simulink model "RBCM_Model"  (R2024b)
settings: Solver=FixedStepAuto  StartTime=0.0  StopTime=10.0  RelTol=1e-3
PreLoadFcn:
  | % NXP_MBDT_S32K3 callback: DO NOT REMOVE
  | mbd_s32k3.common.nxp.model_callbacks.preLoadFcn();
PostLoadFcn:
  | % NXP_MBDT_S32K3 callback: DO NOT REMOVE
  | mbd_s32k3.common.nxp.model_callbacks.postLoadFcn();
InitFcn:
  | % NXP_MBDT_S32K3 callback: DO NOT REMOVE
  | mbd_s32k3.common.nxp.model_callbacks.initFcn();
undefined symbols (not defined in the file or in its folder): AccuFanPwr_hHsd3ch2, BspdPwr_lHsd1ch2, BuzzerPwr_lHsd3ch3, DevicePwr_12v_lHsd1ch1, DevicePwr_hHsd1ch2, DrsPwr_8v_lHsd3ch1, hHsd_Diagnose_AdcBuffer, ILPwr_hHsd1ch1, lHsd_Diagnose_AdcBuffer, LoggerPwr_lHsd1ch3, PumpFan1_hHsd4ch1, PumpFan2_hHsd4ch2, PumpPwr_hHsd3ch1, RGBLED0state, TaillightPwr_lHsd3ch4, TempSensorPwr_lHsd1ch4
libraries: mbd_s32k3_io_library x127, simulink x48, canmsglib x8, mbd_s32k3_communication_library x7, mbd_s32k3_isr_library x6, mbd_s32k3_cdd_library x3, mbd_s32k3_utility_library x1
(part 6 of 10)

== system RBCM_Model/错误码数据发送(未)1 ==
  Trigger : TriggerPort  TriggerType=function-call  VariantControl=(inherit)  PortDimensions=1
  Bus Selector : BusSelector  OutputSignals=Data,Length,ID
  CAN Pack : canmsglib/CAN Pack  CANdbFile=E:\Workspace\Myworkspace\RBCM_S32K344_AUTOSAR_MBD\Firmware\AUTOSAR_MBD\RBCM_ModelConfig\E10_dbc_240819_CAN.dbc  MsgList=RBCM_Diagnose_Data  MsgName=RBCM_Diagnose_Data  MsgIDType=Extended (29-bit identifier)  MsgIdentifier=252996466  CANIDInput=off  MsgLength=2  Remote=off  ApplyMinMax=off  BusOutput=on  SignalInfo={'PDB_Error_Device','0','8','LE','unsigned','Standard','0','1','0','-Inf','Inf';'PDB_Error_State','8','8','LE','unsigned','Standard','0','1','0','-Inf','Inf'}
      settings: LibrarySourceBlock=canlib/CAN Pack  DataFormat=CANdb specified signals
  Can : mbd_s32k3_communication_library/Can  api_func=Can_Write  controller=No controller configured  hw_obj=CanHardwareObject_Can0_Tx_Interrupt  mode=CAN_CS_STARTED  canfd_msg=off  ext_id_msg=off  empty_msg=off  text=|
      | CanConfigSet - CanConfigSet 
      | CanConfigSet/CanController - CanController_0 
      | CanConfigSet/CanController_0/CanAutoBusOffRecovery - false 
      | CanConfigSet/CanController_0/CanBusoffProcessing - POLLING 
      | CanConfigSet/CanController_0/CanControllerActivation - true 
      | CanConfigSet/CanController_0/CanControllerBaseAddress - 0 
      | CanConfigSet/CanController_0/CanControllerBaudrateConfig - CanControllerBaudrateConfig_0 
      | CanConfigSet/CanController_0/CanControllerBaudrateConfig_0/CanAdvancedSetting - false 
      | CanConfigSet/CanController_0/CanControllerBaudrateConfig_0/CanBaudrateTypeSuport - NORMAL_CBT 
      | CanConfigSet/CanController_0/CanControllerBaudrateConfig_0/CanBusLength - 40 
      | CanConfigSet/CanController_0/CanControllerBaudrateConfig_0/CanControllerBaudRate - 500.0 
      | CanConfigSet/CanController_0/CanControllerBaudrateConfig_0/CanControllerBaudRateConfigID - 0 
      | CanConfigSet/CanController_0/CanControllerBaudrateConfig_0/CanControllerFdBaudrateConfig - CanControllerFdBaudrateConfig 
      | CanConfigSet/CanController_0/CanControllerBaudrateConfig_0/CanControllerFdBaudrateConfig/CanControllerFdBaudRate - 2000 
      | CanConfigSet/CanController_0/CanControllerBaudrateConfig_0/CanControllerFdBaudrateConfig/CanControllerFdPrescaller - 2 
      | CanConfigSet/CanController_0/CanControllerBaudrateConfig_0/CanControllerFdBaudrateConfig/CanControllerFdSyncSeg - 1 
      | CanConfigSet/CanController_0/CanControllerBaudrateConfig_0/CanControllerFdBaudrateConfig/CanControllerPrescallerAlternateFd - 1 
      | CanConfigSet/CanController_0/CanControllerBaudrateConfig_0/CanControllerFdBaudrateConfig/CanControllerPropSeg - 5 
      | CanConfigSet/CanController_0/CanControllerBaudrateConfig_0/CanControllerFdBaudrateConfig/CanControllerSeg1 - 2 
      | CanConfigSet/CanController_0/CanControllerBaudrateConfig_0/CanControllerFdBaudrateConfig/CanControllerSeg2 - 2 
      | CanConfigSet/CanController_0/CanControllerBaudrateConfig_0/CanControllerFdBaudrateConfig/CanControllerSyncJumpWidth - 2 
      | CanConfigSet/CanController_0/CanControllerBaudrateConfig_0/CanControllerFdBaudrateConfig/CanControllerTxBitRateSwitch - true 
      | CanConfigSet/CanController_0/CanControllerBaudrateConfig_0/CanControllerFdBaudrateConfig/Index - 0 
      | CanConfigSet/CanController_0/CanControllerBaudrateConfig_0/CanControllerPrescaller - 2 
      | CanConfigSet/CanController_0/CanControllerBaudrateConfig_0/CanControllerPrescallerAlternate - 10 
      | CanConfigSet/CanController_0/CanControllerBaudrateConfig_0/CanControllerPropSeg - 11 
      | CanConfigSet/CanController_0/CanControllerBaudrateConfig_0/CanControllerSeg1 - 18 
      | CanConfigSet/CanController_0/CanControllerBaudrateConfig_0/CanControllerSeg2 - 10 
      | CanConfigSet/CanController_0/CanControllerBaudrateConfig_0/CanControllerSyncJumpWidth - 10 
      | CanConfigSet/CanController_0/CanControllerBaudrateConfig_0/CanControllerSyncSeg - 1 
      | CanConfigSet/CanController_0/CanControllerBaudrateConfig_0/CanPropDelayTranceiver - 150.0 
      | CanConfigSet/CanController_0/CanControllerBaudrateConfig_0/CanTxArbitrationStartDelay - 12 
      | CanConfigSet/CanController_0/CanControllerBaudrateConfig_0/Index - 0 
      | CanConfigSet/CanController_0/CanControllerDefaultBaudrate - /Can_43_FLEXCAN/Can/CanConfigSet/CanController_0/CanControllerBaudrateConfig_0 
      | CanConfigSet/CanController_0/CanControllerEdgeFilter - false 
      | CanConfigSet/CanController_0/CanControllerFdISO - true 
      | CanConfigSet/CanController_0/CanControllerId - 0 
      | CanConfigSet/CanController_0/CanControllerPrExcEn - false 
      | CanConfigSet/CanController_0/CanCpuClockRef - /Mcu/Mcu/McuModuleConfiguration/McuClockSettingConfig_0/FLEXCAN_PE_CLK0_2 
      | CanConfigSet/CanController_0/CanCpuClockRefAlternate - /Mcu/Mcu/McuModuleConfiguration/McuClockSettingConfig_0/FLEXCAN_PE_CLK0_2 
      | CanConfigSet/CanController_0/CanHwChannel - FLEXCAN_0 
      | CanConfigSet/CanController_0/CanLoopBackMode - false 
      | CanConfigSet/CanController_0/CanRamBlock - CanRamBlock 
      | CanConfigSet/CanController_0/CanRamBlock/CanRamBlockUnified - CanRamBlockUnified 
      | CanConfigSet/CanController_0/CanRamBlock/CanRamBlockUnified/CanBlockUnifiedPayloadLength - CAN_16_BYTES_PAYLOAD 
      | CanConfigSet/CanController_0/CanRamBlock/Choice - CanRamBlockUnified 
      | CanConfigSet/CanController_0/CanRamBlock/Index - 0 
      | CanConfigSet/CanController_0/CanRxFiFo - CanRxFiFo 
      | CanConfigSet/CanController_0/CanRxFiFo/CanEnhanceFiFo - CanRxFiFo 
      | CanConfigSet/CanController_0/CanRxFiFo/CanRxFiFo/CanEnhanceFiFoDmaEnable - false 
      | CanConfigSet/CanController_0/CanRxFiFo/CanRxFiFo/CanEnhancedSchemeType - MASK_FILTER_SCHEME 
      | CanConfigSet/CanController_0/CanRxFiFo/CanRxFiFo/CanFiFoDmaErrorNotif - NULL_PTR 
      | CanConfigSet/CanController_0/CanRxFiFo/CanRxFiFo/CanFiFoOverflowNotif - MBDT_FlexCAN0_FifoOverflowNotif 
      | CanConfigSet/CanController_0/CanRxFiFo/CanRxFiFo/NumberMBTransferDMA - 1 
      | CanConfigSet/CanController_0/CanRxFiFo/Choice - CanEnhanceFiFo 
      | CanConfigSet/CanController_0/CanRxFiFo/Index - 0 
      | CanConfigSet/CanController_0/CanRxProcessing - MIXED 
      | CanConfigSet/CanController_0/CanTrippleSamplingEnable - false 
      | CanConfigSet/CanController_0/CanTxProcessing - MIXED 
      | CanConfigSet/CanController_0/CanWakeupFunctionalityAPI - false 
      | CanConfigSet/CanController_0/CanWakeupProcessing - POLLING 
      | CanConfigSet/CanController_0/CanWakeupSupport - false 
      | CanConfigSet/CanController_0/Index - 0 
      | CanConfigSet/CanHardwareObject - CanHardwareObject_Can0_Rx_Ext_Interrupt CanHardwareObject_Can0_Rx_FIFO CanHardwareObject_Can0_Rx_Std_Polling CanHardwareObject_Can0_Tx_Interrupt CanHardwareObject_Can0_Tx_Polling 
      | CanConfigSet/CanHardwareObject_Can0_Rx_Ext_Interrupt/CanControllerRef - /Can_43_FLEXCAN/Can/CanConfigSet/CanController_0 
      | CanConfigSet/CanHardwareObject_Can0_Rx_Ext_Interrupt/CanHandleType - BASIC 
      | CanConfigSet/CanHardwareObject_Can0_Rx_Ext_Interrupt/CanHardwareObjectUsesPolling - false 
      | CanConfigSet/CanHardwareObject_Can0_Rx_Ext_Interrupt/CanHwFilter - CanHwFilter_0 
      | CanConfigSet/CanHardwareObject_Can0_Rx_Ext_Interrupt/CanHwFilter_0/CanHwFilterCode - 0 
      | CanConfigSet/CanHardwareObject_Can0_Rx_Ext_Interrupt/CanHwFilter_0/CanHwFilterMask - 0 
      | CanConfigSet/CanHardwareObject_Can0_Rx_Ext_Interrupt/CanHwFilter_0/Index - 0 
      | CanConfigSet/CanHardwareObject_Can0_Rx_Ext_Interrupt/CanHwObjectCount - 1 
      | CanConfigSet/CanHardwareObject_Can0_Rx_Ext_Interrupt/CanIdType - EXTENDED 
      | CanConfigSet/CanHardwareObject_Can0_Rx_Ext_Interrupt/CanObjectId - 2 
      | CanConfigSet/CanHardwareObject_Can0_Rx_Ext_Interrupt/CanObjectType - RECEIVE 
      | CanConfigSet/CanHardwareObject_Can0_Rx_Ext_Interrupt/Index - 2 
      | CanConfigSet/CanHardwareObject_Can0_Rx_FIFO/CanControllerRef - /Can_43_FLEXCAN/Can/CanConfigSet/CanController_0 
      | CanConfigSet/CanHardwareObject_Can0_Rx_FIFO/CanHandleType - BASIC 
      | CanConfigSet/CanHardwareObject_Can0_Rx_FIFO/CanHardwareObjectUsesPolling - false 
      | CanConfigSet/CanHardwareObject_Can0_Rx_FIFO/CanHwFilter - CanHwFilter_0 CanHwFilter_1 CanHwFilter_2 CanHwFilter_3 CanHwFilter_4 CanHwFilter_5 CanHwFilter_6 CanHwFilter_7 
      | CanConfigSet/CanHardwareObject_Can0_Rx_FIFO/CanHwFilter_0/CanHwFilterCode - 1008 
      | CanConfigSet/CanHardwareObject_Can0_Rx_FIFO/CanHwFilter_0/CanHwFilterMask - 536870911 
      | CanConfigSet/CanHardwareObject_Can0_Rx_FIFO/CanHwFilter_0/Index - 0 
      | CanConfigSet/CanHardwareObject_Can0_Rx_FIFO/CanHwFilter_1/CanHwFilterCode - 1009 
      | CanConfigSet/CanHardwareObject_Can0_Rx_FIFO/CanHwFilter_1/CanHwFilterMask - 536870911 
      | CanConfigSet/CanHardwareObject_Can0_Rx_FIFO/CanHwFilter_1/Index - 1 
      | CanConfigSet/CanHardwareObject_Can0_Rx_FIFO/CanHwFilter_2/CanHwFilterCode - 1010 
      | CanConfigSet/CanHardwareObject_Can0_Rx_FIFO/CanHwFilter_2/CanHwFilterMask - 536870911 
      | CanConfigSet/CanHardwareObject_Can0_Rx_FIFO/CanHwFilter_2/Index - 2 
      | CanConfigSet/CanHardwareObject_Can0_Rx_FIFO/CanHwFilter_3/CanHwFilterCode - 1011 
      | CanConfigSet/CanHardwareObject_Can0_Rx_FIFO/CanHwFilter_3/CanHwFilterMask - 536870911 
      | CanConfigSet/CanHardwareObject_Can0_Rx_FIFO/CanHwFilter_3/Index - 3 
      | CanConfigSet/CanHardwareObject_Can0_Rx_FIFO/CanHwFilter_4/CanHwFilterCode - 1012 
      | CanConfigSet/CanHardwareObject_Can0_Rx_FIFO/CanHwFilter_4/CanHwFilterMask - 536870911 
      | CanConfigSet/CanHardwareObject_Can0_Rx_FIFO/CanHwFilter_4/Index - 4 
      | CanConfigSet/CanHardwareObject_Can0_Rx_FIFO/CanHwFilter_5/CanHwFilterCode - 1013 
      | CanConfigSet/CanHardwareObject_Can0_Rx_FIFO/CanHwFilter_5/CanHwFilterMask - 536870911 
      | CanConfigSet/CanHardwareObject_Can0_Rx_FIFO/CanHwFilter_5/Index - 5 
      | CanConfigSet/CanHardwareObject_Can0_Rx_FIFO/CanHwFilter_6/CanHwFilterCode - 1014 
      | CanConfigSet/CanHardwareObject_Can0_Rx_FIFO/CanHwFilter_6/CanHwFilterMask - 536870911 
      | CanConfigSet/CanHardwareObject_Can0_Rx_FIFO/CanHwFilter_6/Index - 6 
      | CanConfigSet/CanHardwareObject_Can0_Rx_FIFO/CanHwFilter_7/CanHwFilterCode - 1015 
      | CanConfigSet/CanHardwareObject_Can0_Rx_FIFO/CanHwFilter_7/CanHwFilterMask - 536870911 
      | CanConfigSet/CanHardwareObject_Can0_Rx_FIFO/CanHwFilter_7/Index - 7 
      | CanConfigSet/CanHardwareObject_Can0_Rx_FIFO/CanHwObjectCount - 6 
      | CanConfigSet/CanHardwareObject_Can0_Rx_FIFO/CanIdType - EXTENDED 
      | CanConfigSet/CanHardwareObject_Can0_Rx_FIFO/CanObjectId - 0 
      | CanConfigSet/CanHardwareObject_Can0_Rx_FIFO/CanObjectType - RECEIVE 
      | CanConfigSet/CanHardwareObject_Can0_Rx_FIFO/Index - 0 
      | CanConfigSet/CanHardwareObject_Can0_Rx_Std_Polling/CanControllerRef - /Can_43_FLEXCAN/Can/CanConfigSet/CanController_0 
      | CanConfigSet/CanHardwareObject_Can0_Rx_Std_Polling/CanHandleType - BASIC 
      | CanConfigSet/CanHardwareObject_Can0_Rx_Std_Polling/CanHardwareObjectUsesPolling - true 
      | CanConfigSet/CanHardwareObject_Can0_Rx_Std_Polling/CanHwFilter - CanHwFilter_0 
      | CanConfigSet/CanHardwareObject_Can0_Rx_Std_Polling/CanHwFilter_0/CanHwFilterCode - 0 
      | CanConfigSet/CanHardwareObject_Can0_Rx_Std_Polling/CanHwFilter_0/CanHwFilterMask - 0 
      | CanConfigSet/CanHardwareObject_Can0_Rx_Std_Polling/CanHwFilter_0/Index - 0 
      | CanConfigSet/CanHardwareObject_Can0_Rx_Std_Polling/CanHwObjectCount - 1 
      | CanConfigSet/CanHardwareObject_Can0_Rx_Std_Polling/CanIdType - STANDARD 
      | CanConfigSet/CanHardwareObject_Can0_Rx_Std_Polling/CanMainFunctionRWPeriodRef - /Can_43_FLEXCAN/Can/CanGeneral/CanMainFunctionRWPeriods_0 
      | CanConfigSet/CanHardwareObject_Can0_Rx_Std_Polling/CanObjectId - 1 
      | CanConfigSet/CanHardwareObject_Can0_Rx_Std_Polling/CanObjectType - RECEIVE 
      | CanConfigSet/CanHardwareObject_Can0_Rx_Std_Polling/Index - 1 
      | CanConfigSet/CanHardwareObject_Can0_Tx_Interrupt/CanControllerRef - /Can_43_FLEXCAN/Can/CanConfigSet/CanController_0 
      | CanConfigSet/CanHardwareObject_Can0_Tx_Interrupt/CanHandleType - BASIC 
      | CanConfigSet/CanHardwareObject_Can0_Tx_Interrupt/CanHardwareObjectUsesPolling - false 
      | CanConfigSet/CanHardwareObject_Can0_Tx_Interrupt/CanHwObjectCount - 1 
      | CanConfigSet/CanHardwareObject_Can0_Tx_Interrupt/CanIdType - MIXED 
      | CanConfigSet/CanHardwareObject_Can0_Tx_Interrupt/CanObjectId - 4 
      | CanConfigSet/CanHardwareObject_Can0_Tx_Interrupt/CanObjectType - TRANSMIT 
      | CanConfigSet/CanHardwareObject_Can0_Tx_Interrupt/Index - 4 
      | CanConfigSet/CanHardwareObject_Can0_Tx_Polling/CanControllerRef - /Can_43_FLEXCAN/Can/CanConfigSet/CanController_0 
      | CanConfigSet/CanHardwareObject_Can0_Tx_Polling/CanHandleType - BASIC 
      | CanConfigSet/CanHardwareObject_Can0_Tx_Polling/CanHardwareObjectUsesPolling - true 
      | CanConfigSet/CanHardwareObject_Can0_Tx_Polling/CanHwObjectCount - 1 
      | CanConfigSet/CanHardwareObject_Can0_Tx_Polling/CanIdType - MIXED 
      | CanConfigSet/CanHardwareObject_Can0_Tx_Polling/CanMainFunctionRWPeriodRef - /Can_43_FLEXCAN/Can/CanGeneral/CanMainFunctionRWPeriods_0 
      | CanConfigSet/CanHardwareObject_Can0_Tx_Polling/CanObjectId - 3 
      | CanConfigSet/CanHardwareObject_Can0_Tx_Polling/CanObjectType - TRANSMIT 
      | CanConfigSet/CanHardwareObject_Can0_Tx_Polling/Index - 3 
      | CanGeneral - CanGeneral 
      | CanGeneral/CanApiEnableMbAbort - true 
      | CanGeneral/CanDevErrorDetect - true 
      | CanGeneral/CanEnableDualClockMode - false 
      | CanGeneral/CanEnableSecurityEventReporting - false 
      | CanGeneral/CanEnableUserModeSupport - false 
      | CanGeneral/CanGlobalTimeSupport - false 
      | CanGeneral/CanIndex - 0 
      | CanGeneral/CanMBCountExtensionSupport - false 
      | CanGeneral/CanMainFunctionModePeriod - 0.001 
      | CanGeneral/CanMainFunctionRWPeriods - CanMainFunctionRWPeriods_0 
      | CanGeneral/CanMainFunctionRWPeriods_0/CanMainFunctionPeriod - 0.001 
      | CanGeneral/CanMainFunctionRWPeriods_0/Index - 0 
      | CanGeneral/CanMultiPartitionSupport - false 
      | CanGeneral/CanMultiplexedTransmission - true 
      | CanGeneral/CanSetBaudrateApi - true 
      | CanGeneral/CanTimeoutDuration - 1.0 
      | CanGeneral/CanTimeoutMethod - OSIF_COUNTER_DUMMY 
      | CanGeneral/CanVersionInfoApi - true 
      | CommonPublishedInformation - CommonPublishedInformation 
      | CommonPublishedInformation/ArReleaseMajorVersion - 4 
      | CommonPublishedInformation/ArReleaseMinorVersion - 7 
      | CommonPublishedInformation/ArReleaseRevisionVersion - 0 
      | CommonPublishedInformation/ModuleId - 80 
      | CommonPublishedInformation/SwMajorVersion - 3 
      | CommonPublishedInformation/SwMinorVersion - 0 
      | CommonPublishedInformation/SwPatchVersion - 0 
      | CommonPublishedInformation/VendorApiInfix - FLEXCAN 
      | CommonPublishedInformation/VendorId - 43 
      | IMPLEMENTATION-CONFIG-VARIANT - VARIANT-POST-BUILD 
      | POST_BUILD_VARIANT_USED - true
      settings: SourceProductName=Communication Blocks
  Constant : Constant  Value=0  OutDataTypeStr=uint16
  Constant2 : Constant  OutDataTypeStr=uint8
  Constant3 : Constant  OutDataTypeStr=uint8
  Data Store Write1 : DataStoreWrite  DataStoreName=can_id  IndexOptions=Index vector (dialog)  Indices=1  OutputSizes=1
  Terminator : Terminator
  Terminator2 : Terminator
  wires:
  Constant/1 -> Can/2
  Constant3/1 -> CAN Pack/2
  Constant2/1 -> CAN Pack/1
  Can/1 -> Terminator/1
  Bus Selector/1 -> Can/3  "<Data>"
  CAN Pack/1 -> Bus Selector/1
  Bus Selector/3 -> Data Store Write1/1, Can/1  "<ID>"
  Bus Selector/2 -> Terminator2/1  "<Length>"

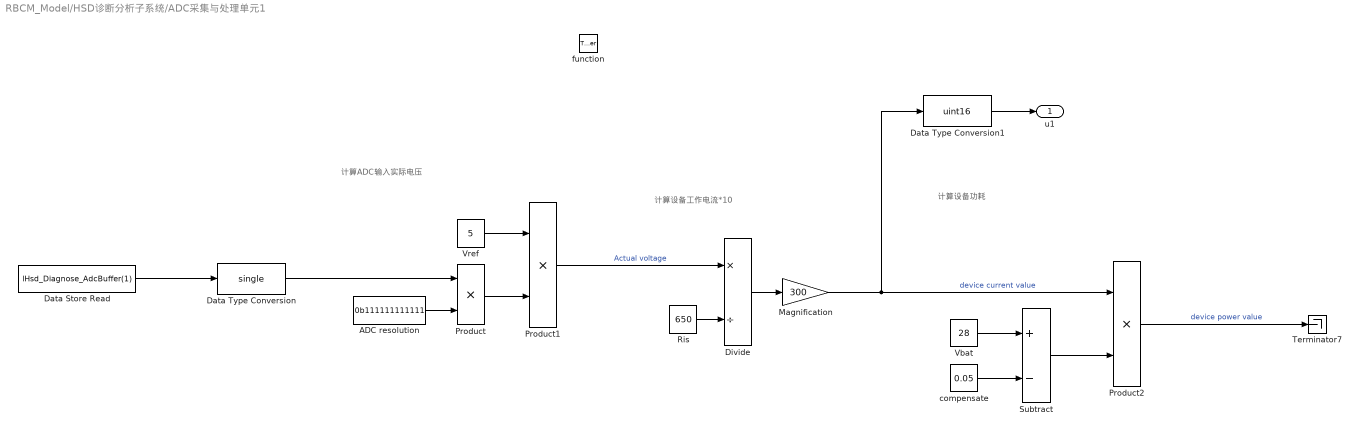
== system RBCM_Model/HSD诊断分析子系统/ADC采集与处理单元1 ==
  note: 计算设备功耗
  note: 计算设备工作电流*10
  note: 计算ADC输入实际电压
  function : TriggerPort  TriggerType=function-call  VariantControl=Variant
  ADC resolution : Constant  Value=0b111111111111  OutDataTypeStr=uint16
  Data Store Read : DataStoreRead  DataStoreName=lHsd_Diagnose_AdcBuffer  DataStoreElements=lHsd_Diagnose_AdcBuffer(1)  IndexOptions=Index vector (dialog)  Indices=1  OutputSizes=1
  Data Type Conversion : DataTypeConversion  OutDataTypeStr=single  SaturateOnIntegerOverflow=off  RndMeth=Floor
  Data Type Conversion1 : DataTypeConversion  OutDataTypeStr=uint16  SaturateOnIntegerOverflow=off  RndMeth=Floor
  Divide : Product  Inputs=*/  OutDataTypeStr=single
  Magnification : Gain  Gain=300
  Product : Product  OutDataTypeStr=single
  Product1 : Product  OutDataTypeStr=single
  Product2 : Product  OutDataTypeStr=single
  Ris : Constant  Value=650  OutDataTypeStr=uint16
  Subtract : Sum  Inputs=+-
  Terminator7 : Terminator
  Vbat : Constant  Value=28  OutDataTypeStr=uint16
  Vref : Constant  Value=5  OutDataTypeStr=uint8
  compensate : Constant  Value=0.05  OutDataTypeStr=single
  u1 : Outport
  wires:
  Magnification/1 -> Data Type Conversion1/1, Product2/1  "device current value"
  Divide/1 -> Magnification/1
  Ris/1 -> Divide/2
  Product1/1 -> Divide/1  "Actual voltage"
  Vref/1 -> Product1/1
  Product/1 -> Product1/2
  ADC resolution/1 -> Product/2
  Data Store Read/1 -> Data Type Conversion/1
  Vbat/1 -> Subtract/1
  compensate/1 -> Subtract/2
  Subtract/1 -> Product2/2
  Product2/1 -> Terminator7/1  "device power value"
  Data Type Conversion/1 -> Product/1
  Data Type Conversion1/1 -> u1/1

== system RBCM_Model/HSD诊断分析子系统/ADC采集与处理单元10 ==
  note: 计算设备功耗
  note: 计算ADC输入实际电压
  note: 计算设备工作电流
  function : TriggerPort  TriggerType=function-call  VariantControl=Variant
  ADC resolution : Constant  Value=0b111111111111  OutDataTypeStr=uint16
  Data Store Read : DataStoreRead  DataStoreName=hHsd_Diagnose_AdcBuffer  DataStoreElements=hHsd_Diagnose_AdcBuffer(1)  IndexOptions=Index vector (dialog)  Indices=1  OutputSizes=1
  Data Type Conversion : DataTypeConversion  OutDataTypeStr=single  SaturateOnIntegerOverflow=off  RndMeth=Floor
  Data Type Conversion1 : DataTypeConversion  OutDataTypeStr=uint16  SaturateOnIntegerOverflow=off  RndMeth=Floor
  Divide : Product  Inputs=*/  OutDataTypeStr=single
  Magnification : Gain  Gain=1450
  Product : Product  OutDataTypeStr=single
  Product1 : Product  OutDataTypeStr=single
  Product2 : Product  OutDataTypeStr=single
  Ris : Constant  Value=650  OutDataTypeStr=uint16
  Subtract : Sum  Inputs=+-
  Terminator7 : Terminator
  Vbat : Constant  Value=28  OutDataTypeStr=uint16
  Vref : Constant  Value=5  OutDataTypeStr=uint8
  compensate : Constant  Value=0.05  OutDataTypeStr=single
  u : Outport
  wires:
  Data Type Conversion1/1 -> u/1
  Magnification/1 -> Product2/1, Data Type Conversion1/1  "device current value"
  ADC resolution/1 -> Product/2
  Ris/1 -> Divide/2
  Divide/1 -> Magnification/1
  Subtract/1 -> Product2/2
  Vref/1 -> Product1/1
  Product/1 -> Product1/2
  Vbat/1 -> Subtract/1
  Product1/1 -> Divide/1  "Actual voltage"
  compensate/1 -> Subtract/2
  Product2/1 -> Terminator7/1  "device power value"
  Data Type Conversion/1 -> Product/1
  Data Store Read/1 -> Data Type Conversion/1

== system RBCM_Model/HSD诊断分析子系统/ADC采集与处理单元11 ==
  note: 计算设备工作电流
  note: 计算ADC输入实际电压
  note: 计算设备功耗
  function : TriggerPort  TriggerType=function-call  VariantControl=Variant
  ADC resolution : Constant  Value=0b111111111111  OutDataTypeStr=uint16
  Data Store Read : DataStoreRead  DataStoreName=hHsd_Diagnose_AdcBuffer  DataStoreElements=hHsd_Diagnose_AdcBuffer(1)  IndexOptions=Index vector (dialog)  Indices=1  OutputSizes=1
  Data Type Conversion : DataTypeConversion  OutDataTypeStr=single  SaturateOnIntegerOverflow=off  RndMeth=Floor
  Data Type Conversion1 : DataTypeConversion  OutDataTypeStr=uint16  SaturateOnIntegerOverflow=off  RndMeth=Floor
  Divide : Product  Inputs=*/  OutDataTypeStr=single
  Magnification : Gain  Gain=1450
  Product : Product  OutDataTypeStr=single
  Product1 : Product  OutDataTypeStr=single
  Product2 : Product  OutDataTypeStr=single
  Ris : Constant  Value=650  OutDataTypeStr=uint16
  Subtract : Sum  Inputs=+-
  Terminator7 : Terminator
  Vbat : Constant  Value=28  OutDataTypeStr=uint16
  Vref : Constant  Value=5  OutDataTypeStr=uint8
  compensate : Constant  Value=0.05  OutDataTypeStr=single
  u : Outport
  wires:
  Data Store Read/1 -> Data Type Conversion/1
  Data Type Conversion/1 -> Product/1
  Product2/1 -> Terminator7/1  "device power value"
  compensate/1 -> Subtract/2
  Product1/1 -> Divide/1  "Actual voltage"
  Vbat/1 -> Subtract/1
  Product/1 -> Product1/2
  Vref/1 -> Product1/1
  Subtract/1 -> Product2/2
  Divide/1 -> Magnification/1
  Ris/1 -> Divide/2
  ADC resolution/1 -> Product/2
  Magnification/1 -> Data Type Conversion1/1, Product2/1  "device current value"
  Data Type Conversion1/1 -> u/1

== system RBCM_Model/HSD诊断分析子系统/ADC采集与处理单元2 ==
  note: 计算设备功耗
  note: 计算设备工作电流*10
  note: 计算ADC输入实际电压
  function : TriggerPort  TriggerType=function-call  VariantControl=Variant
  ADC resolution : Constant  Value=0b111111111111  OutDataTypeStr=uint16
  Data Store Read : DataStoreRead  DataStoreName=lHsd_Diagnose_AdcBuffer  DataStoreElements=lHsd_Diagnose_AdcBuffer(1)  IndexOptions=Index vector (dialog)  Indices=1  OutputSizes=1
  Data Type Conversion : DataTypeConversion  OutDataTypeStr=single  SaturateOnIntegerOverflow=off  RndMeth=Floor
  Data Type Conversion1 : DataTypeConversion  OutDataTypeStr=uint16  SaturateOnIntegerOverflow=off  RndMeth=Floor
  Divide : Product  Inputs=*/  OutDataTypeStr=single
  Magnification : Gain  Gain=300
  Product : Product  OutDataTypeStr=single
  Product1 : Product  OutDataTypeStr=single
  Product2 : Product  OutDataTypeStr=single
  Ris : Constant  Value=650  OutDataTypeStr=uint16
  Subtract : Sum  Inputs=+-
  Terminator7 : Terminator
  Vbat : Constant  Value=28  OutDataTypeStr=uint16
  Vref : Constant  Value=5  OutDataTypeStr=uint8
  compensate : Constant  Value=0.05  OutDataTypeStr=single
  u1 : Outport
  wires:
  Magnification/1 -> Data Type Conversion1/1, Product2/1  "device current value"
  Divide/1 -> Magnification/1
  Ris/1 -> Divide/2
  Product1/1 -> Divide/1  "Actual voltage"
  Vref/1 -> Product1/1
  Product/1 -> Product1/2
  ADC resolution/1 -> Product/2
  Data Store Read/1 -> Data Type Conversion/1
  Vbat/1 -> Subtract/1
  compensate/1 -> Subtract/2
  Subtract/1 -> Product2/2
  Product2/1 -> Terminator7/1  "device power value"
  Data Type Conversion/1 -> Product/1
  Data Type Conversion1/1 -> u1/1

== system RBCM_Model/HSD诊断分析子系统/ADC采集与处理单元3 ==
  note: 计算ADC输入实际电压
  note: 计算设备工作电流*10
  note: 计算设备功耗
  function : TriggerPort  TriggerType=function-call  VariantControl=Variant
  ADC resolution : Constant  Value=0b111111111111  OutDataTypeStr=uint16
  Data Store Read : DataStoreRead  DataStoreName=lHsd_Diagnose_AdcBuffer  DataStoreElements=lHsd_Diagnose_AdcBuffer(1)  IndexOptions=Index vector (dialog)  Indices=1  OutputSizes=1
  Data Type Conversion : DataTypeConversion  OutDataTypeStr=single  SaturateOnIntegerOverflow=off  RndMeth=Floor
  Data Type Conversion1 : DataTypeConversion  OutDataTypeStr=uint16  SaturateOnIntegerOverflow=off  RndMeth=Floor
  Divide : Product  Inputs=*/  OutDataTypeStr=single
  Magnification : Gain  Gain=300
  Product : Product  OutDataTypeStr=single
  Product1 : Product  OutDataTypeStr=single
  Product2 : Product  OutDataTypeStr=single
  Ris : Constant  Value=650  OutDataTypeStr=uint16
  Subtract : Sum  Inputs=+-
  Terminator7 : Terminator
  Vbat : Constant  Value=28  OutDataTypeStr=uint16
  Vref : Constant  Value=5  OutDataTypeStr=uint8
  compensate : Constant  Value=0.05  OutDataTypeStr=single
  u1 : Outport
  wires:
  Data Type Conversion1/1 -> u1/1
  Data Type Conversion/1 -> Product/1
  Product2/1 -> Terminator7/1  "device power value"
  Subtract/1 -> Product2/2
  compensate/1 -> Subtract/2
  Vbat/1 -> Subtract/1
  Data Store Read/1 -> Data Type Conversion/1
  ADC resolution/1 -> Product/2
  Product/1 -> Product1/2
  Vref/1 -> Product1/1
  Product1/1 -> Divide/1  "Actual voltage"
  Ris/1 -> Divide/2
  Divide/1 -> Magnification/1
  Magnification/1 -> Product2/1, Data Type Conversion1/1  "device current value"

== system RBCM_Model/HSD诊断分析子系统/ADC采集与处理单元4 ==
  note: 计算设备功耗
  note: 计算设备工作电流*10
  note: 计算ADC输入实际电压
  function : TriggerPort  TriggerType=function-call  VariantControl=Variant
  ADC resolution : Constant  Value=0b111111111111  OutDataTypeStr=uint16
  Data Store Read : DataStoreRead  DataStoreName=lHsd_Diagnose_AdcBuffer  DataStoreElements=lHsd_Diagnose_AdcBuffer(1)  IndexOptions=Index vector (dialog)  Indices=1  OutputSizes=1
  Data Type Conversion : DataTypeConversion  OutDataTypeStr=single  SaturateOnIntegerOverflow=off  RndMeth=Floor
  Data Type Conversion1 : DataTypeConversion  OutDataTypeStr=uint16  SaturateOnIntegerOverflow=off  RndMeth=Floor
  Divide : Product  Inputs=*/  OutDataTypeStr=single
  Magnification : Gain  Gain=300
  Product : Product  OutDataTypeStr=single
  Product1 : Product  OutDataTypeStr=single
  Product2 : Product  OutDataTypeStr=single
  Ris : Constant  Value=650  OutDataTypeStr=uint16
  Subtract : Sum  Inputs=+-
  Terminator7 : Terminator
  Vbat : Constant  Value=28  OutDataTypeStr=uint16
  Vref : Constant  Value=5  OutDataTypeStr=uint8
  compensate : Constant  Value=0.05  OutDataTypeStr=single
  u1 : Outport
  wires:
  Magnification/1 -> Data Type Conversion1/1, Product2/1  "device current value"
  Divide/1 -> Magnification/1
  Ris/1 -> Divide/2
  Product1/1 -> Divide/1  "Actual voltage"
  Vref/1 -> Product1/1
  Product/1 -> Product1/2
  ADC resolution/1 -> Product/2
  Data Store Read/1 -> Data Type Conversion/1
  Vbat/1 -> Subtract/1
  compensate/1 -> Subtract/2
  Subtract/1 -> Product2/2
  Product2/1 -> Terminator7/1  "device power value"
  Data Type Conversion/1 -> Product/1
  Data Type Conversion1/1 -> u1/1

== system RBCM_Model/HSD诊断分析子系统/ADC采集与处理单元5 ==
  note: 计算ADC输入实际电压
  note: 计算设备工作电流*10
  note: 计算设备功耗
  function : TriggerPort  TriggerType=function-call  VariantControl=Variant
  ADC resolution : Constant  Value=0b111111111111  OutDataTypeStr=uint16
  Data Store Read : DataStoreRead  DataStoreName=lHsd_Diagnose_AdcBuffer  DataStoreElements=lHsd_Diagnose_AdcBuffer(1)  IndexOptions=Index vector (dialog)  Indices=1  OutputSizes=1
  Data Type Conversion : DataTypeConversion  OutDataTypeStr=single  SaturateOnIntegerOverflow=off  RndMeth=Floor
  Data Type Conversion1 : DataTypeConversion  OutDataTypeStr=uint16  SaturateOnIntegerOverflow=off  RndMeth=Floor
  Divide : Product  Inputs=*/  OutDataTypeStr=single
  Magnification : Gain  Gain=300
  Product : Product  OutDataTypeStr=single
  Product1 : Product  OutDataTypeStr=single
  Product2 : Product  OutDataTypeStr=single
  Ris : Constant  Value=650  OutDataTypeStr=uint16
  Subtract : Sum  Inputs=+-
  Terminator7 : Terminator
  Vbat : Constant  Value=28  OutDataTypeStr=uint16
  Vref : Constant  Value=5  OutDataTypeStr=uint8
  compensate : Constant  Value=0.05  OutDataTypeStr=single
  u1 : Outport
  wires:
  Data Type Conversion1/1 -> u1/1
  Data Type Conversion/1 -> Product/1
  Product2/1 -> Terminator7/1  "device power value"
  Subtract/1 -> Product2/2
  compensate/1 -> Subtract/2
  Vbat/1 -> Subtract/1
  Data Store Read/1 -> Data Type Conversion/1
  ADC resolution/1 -> Product/2
  Product/1 -> Product1/2
  Vref/1 -> Product1/1
  Product1/1 -> Divide/1  "Actual voltage"
  Ris/1 -> Divide/2
  Divide/1 -> Magnification/1
  Magnification/1 -> Product2/1, Data Type Conversion1/1  "device current value"

== system RBCM_Model/HSD诊断分析子系统/ADC采集与处理单元6 ==
  note: 计算设备功耗
  note: 计算ADC输入实际电压
  note: 计算设备工作电流
  function : TriggerPort  TriggerType=function-call  VariantControl=Variant
  ADC resolution : Constant  Value=0b111111111111  OutDataTypeStr=uint16
  Data Store Read : DataStoreRead  DataStoreName=hHsd_Diagnose_AdcBuffer  DataStoreElements=hHsd_Diagnose_AdcBuffer(1)  IndexOptions=Index vector (dialog)  Indices=1  OutputSizes=1
  Data Type Conversion : DataTypeConversion  OutDataTypeStr=single  SaturateOnIntegerOverflow=off  RndMeth=Floor
  Data Type Conversion1 : DataTypeConversion  OutDataTypeStr=uint16  SaturateOnIntegerOverflow=off  RndMeth=Floor
  Divide : Product  Inputs=*/  OutDataTypeStr=single
  Magnification : Gain  Gain=1450
  Product : Product  OutDataTypeStr=single
  Product1 : Product  OutDataTypeStr=single
  Product2 : Product  OutDataTypeStr=single
  Ris : Constant  Value=650  OutDataTypeStr=uint16
  Subtract : Sum  Inputs=+-
  Terminator7 : Terminator
  Vbat : Constant  Value=28  OutDataTypeStr=uint16
  Vref : Constant  Value=5  OutDataTypeStr=uint8
  compensate : Constant  Value=0.05  OutDataTypeStr=single
  u : Outport
  wires:
  Data Type Conversion1/1 -> u/1
  Magnification/1 -> Product2/1, Data Type Conversion1/1  "device current value"
  ADC resolution/1 -> Product/2
  Ris/1 -> Divide/2
  Divide/1 -> Magnification/1
  Subtract/1 -> Product2/2
  Vref/1 -> Product1/1
  Product/1 -> Product1/2
  Vbat/1 -> Subtract/1
  Product1/1 -> Divide/1  "Actual voltage"
  compensate/1 -> Subtract/2
  Product2/1 -> Terminator7/1  "device power value"
  Data Type Conversion/1 -> Product/1
  Data Store Read/1 -> Data Type Conversion/1

== system RBCM_Model/HSD诊断分析子系统/ADC采集与处理单元7 ==
  note: 计算设备工作电流
  note: 计算ADC输入实际电压
  note: 计算设备功耗
  function : TriggerPort  TriggerType=function-call  VariantControl=Variant
  ADC resolution : Constant  Value=0b111111111111  OutDataTypeStr=uint16
  Data Store Read : DataStoreRead  DataStoreName=hHsd_Diagnose_AdcBuffer  DataStoreElements=hHsd_Diagnose_AdcBuffer(1)  IndexOptions=Index vector (dialog)  Indices=1  OutputSizes=1
  Data Type Conversion : DataTypeConversion  OutDataTypeStr=single  SaturateOnIntegerOverflow=off  RndMeth=Floor
  Data Type Conversion1 : DataTypeConversion  OutDataTypeStr=uint16  SaturateOnIntegerOverflow=off  RndMeth=Floor
  Divide : Product  Inputs=*/  OutDataTypeStr=single
  Magnification : Gain  Gain=1450
  Product : Product  OutDataTypeStr=single
  Product1 : Product  OutDataTypeStr=single
  Product2 : Product  OutDataTypeStr=single
  Ris : Constant  Value=650  OutDataTypeStr=uint16
  Subtract : Sum  Inputs=+-
  Terminator7 : Terminator
  Vbat : Constant  Value=28  OutDataTypeStr=uint16
  Vref : Constant  Value=5  OutDataTypeStr=uint8
  compensate : Constant  Value=0.05  OutDataTypeStr=single
  u : Outport
  wires:
  Data Store Read/1 -> Data Type Conversion/1
  Data Type Conversion/1 -> Product/1
  Product2/1 -> Terminator7/1  "device power value"
  compensate/1 -> Subtract/2
  Product1/1 -> Divide/1  "Actual voltage"
  Vbat/1 -> Subtract/1
  Product/1 -> Product1/2
  Vref/1 -> Product1/1
  Subtract/1 -> Product2/2
  Divide/1 -> Magnification/1
  Ris/1 -> Divide/2
  ADC resolution/1 -> Product/2
  Magnification/1 -> Data Type Conversion1/1, Product2/1  "device current value"
  Data Type Conversion1/1 -> u/1

== system RBCM_Model/HSD诊断分析子系统/ADC采集与处理单元8 ==
  note: 计算设备功耗
  note: 计算ADC输入实际电压
  note: 计算设备工作电流
  function : TriggerPort  TriggerType=function-call  VariantControl=Variant
  ADC resolution : Constant  Value=0b111111111111  OutDataTypeStr=uint16
  Data Store Read : DataStoreRead  DataStoreName=hHsd_Diagnose_AdcBuffer  DataStoreElements=hHsd_Diagnose_AdcBuffer(1)  IndexOptions=Index vector (dialog)  Indices=1  OutputSizes=1
  Data Type Conversion : DataTypeConversion  OutDataTypeStr=single  SaturateOnIntegerOverflow=off  RndMeth=Floor
  Data Type Conversion1 : DataTypeConversion  OutDataTypeStr=uint16  SaturateOnIntegerOverflow=off  RndMeth=Floor
  Divide : Product  Inputs=*/  OutDataTypeStr=single
  Magnification : Gain  Gain=1450
  Product : Product  OutDataTypeStr=single
  Product1 : Product  OutDataTypeStr=single
  Product2 : Product  OutDataTypeStr=single
  Ris : Constant  Value=650  OutDataTypeStr=uint16
  Subtract : Sum  Inputs=+-
  Terminator7 : Terminator
  Vbat : Constant  Value=28  OutDataTypeStr=uint16
  Vref : Constant  Value=5  OutDataTypeStr=uint8
  compensate : Constant  Value=0.05  OutDataTypeStr=single
  u : Outport
  wires:
  Data Type Conversion1/1 -> u/1
  Magnification/1 -> Product2/1, Data Type Conversion1/1  "device current value"
  ADC resolution/1 -> Product/2
  Ris/1 -> Divide/2
  Divide/1 -> Magnification/1
  Subtract/1 -> Product2/2
  Vref/1 -> Product1/1
  Product/1 -> Product1/2
  Vbat/1 -> Subtract/1
  Product1/1 -> Divide/1  "Actual voltage"
  compensate/1 -> Subtract/2
  Product2/1 -> Terminator7/1  "device power value"
  Data Type Conversion/1 -> Product/1
  Data Store Read/1 -> Data Type Conversion/1

== system RBCM_Model/HSD诊断分析子系统/ADC采集与处理单元9 ==
  note: 计算设备工作电流
  note: 计算ADC输入实际电压
  note: 计算设备功耗
  function : TriggerPort  TriggerType=function-call  VariantControl=Variant
  ADC resolution : Constant  Value=0b111111111111  OutDataTypeStr=uint16
  Data Store Read : DataStoreRead  DataStoreName=hHsd_Diagnose_AdcBuffer  DataStoreElements=hHsd_Diagnose_AdcBuffer(1)  IndexOptions=Index vector (dialog)  Indices=1  OutputSizes=1
  Data Type Conversion : DataTypeConversion  OutDataTypeStr=single  SaturateOnIntegerOverflow=off  RndMeth=Floor
  Data Type Conversion1 : DataTypeConversion  OutDataTypeStr=uint16  SaturateOnIntegerOverflow=off  RndMeth=Floor
  Divide : Product  Inputs=*/  OutDataTypeStr=single
  Magnification : Gain  Gain=1450
  Product : Product  OutDataTypeStr=single
  Product1 : Product  OutDataTypeStr=single
  Product2 : Product  OutDataTypeStr=single
  Ris : Constant  Value=650  OutDataTypeStr=uint16
  Subtract : Sum  Inputs=+-
  Terminator7 : Terminator
  Vbat : Constant  Value=28  OutDataTypeStr=uint16
  Vref : Constant  Value=5  OutDataTypeStr=uint8
  compensate : Constant  Value=0.05  OutDataTypeStr=single
  u : Outport
  wires:
  Data Store Read/1 -> Data Type Conversion/1
  Data Type Conversion/1 -> Product/1
  Product2/1 -> Terminator7/1  "device power value"
  compensate/1 -> Subtract/2
  Product1/1 -> Divide/1  "Actual voltage"
  Vbat/1 -> Subtract/1
  Product/1 -> Product1/2
  Vref/1 -> Product1/1
  Subtract/1 -> Product2/2
  Divide/1 -> Magnification/1
  Ris/1 -> Divide/2
  ADC resolution/1 -> Product/2
  Magnification/1 -> Data Type Conversion1/1, Product2/1  "device current value"
  Data Type Conversion1/1 -> u/1

== system RBCM_Model/HSD诊断分析子系统/HSDh片选执行单元1 ==
  y : Inport
  Data Type Conversion4 : DataTypeConversion  OutDataTypeStr=uint8  SaturateOnIntegerOverflow=off  RndMeth=Floor
  Dio : mbd_s32k3_io_library/Dio  Commented=on  api_func=Dio_WriteChannel  channel=RGBLED0_BLUE  channel_group=No channel groups configured  port=PTB_H  gpioSim=on  text=<binary blob, 15399 chars, not shown>
      settings: SourceProductName=IO Blocks
  wires:
  Data Type Conversion4/1 -> Dio/1
  y/1 -> Data Type Conversion4/1

== system RBCM_Model/HSD诊断分析子系统/HSDh片选执行单元11 ==
  y : Inport
  Data Type Conversion4 : DataTypeConversion  OutDataTypeStr=uint8  SaturateOnIntegerOverflow=off  RndMeth=Floor
  Dio : mbd_s32k3_io_library/Dio  api_func=Dio_WriteChannel  channel=RGBLED0_BLUE  channel_group=No channel groups configured  port=PTB_H  gpioSim=on  text=<binary blob, 15399 chars, not shown>
      settings: SourceProductName=IO Blocks
  wires:
  y/1 -> Data Type Conversion4/1
  Data Type Conversion4/1 -> Dio/1

== system RBCM_Model/HSD诊断分析子系统/HSDh片选执行单元2 ==
  y : Inport
  Data Type Conversion4 : DataTypeConversion  OutDataTypeStr=uint8  SaturateOnIntegerOverflow=off  RndMeth=Floor
  Dio : mbd_s32k3_io_library/Dio  api_func=Dio_WriteChannel  channel=RGBLED0_BLUE  channel_group=No channel groups configured  port=PTB_H  gpioSim=on  text=<binary blob, 15399 chars, not shown>
      settings: SourceProductName=IO Blocks
  wires:
  y/1 -> Data Type Conversion4/1
  Data Type Conversion4/1 -> Dio/1

== system RBCM_Model/HSD诊断分析子系统/HSDh片选执行单元3 ==
  y : Inport
  Data Type Conversion4 : DataTypeConversion  OutDataTypeStr=uint8  SaturateOnIntegerOverflow=off  RndMeth=Floor
  Dio : mbd_s32k3_io_library/Dio  api_func=Dio_WriteChannel  channel=RGBLED0_BLUE  channel_group=No channel groups configured  port=PTB_H  gpioSim=on  text=<binary blob, 15399 chars, not shown>
      settings: SourceProductName=IO Blocks
  wires:
  Data Type Conversion4/1 -> Dio/1
  y/1 -> Data Type Conversion4/1

== system RBCM_Model/HSD诊断分析子系统/HSDh片选执行单元4 ==
  y : Inport
  Data Type Conversion4 : DataTypeConversion  OutDataTypeStr=uint8  SaturateOnIntegerOverflow=off  RndMeth=Floor
  Dio : mbd_s32k3_io_library/Dio  api_func=Dio_WriteChannel  channel=RGBLED0_BLUE  channel_group=No channel groups configured  port=PTB_H  gpioSim=on  text=<binary blob, 15399 chars, not shown>
      settings: SourceProductName=IO Blocks
  wires:
  Data Type Conversion4/1 -> Dio/1
  y/1 -> Data Type Conversion4/1

== system RBCM_Model/HSD诊断分析子系统/HSDh片选执行单元5 ==
  y : Inport
  Data Type Conversion4 : DataTypeConversion  OutDataTypeStr=uint8  SaturateOnIntegerOverflow=off  RndMeth=Floor
  Dio : mbd_s32k3_io_library/Dio  api_func=Dio_WriteChannel  channel=RGBLED0_BLUE  channel_group=No channel groups configured  port=PTB_H  gpioSim=on  text=<binary blob, 15399 chars, not shown>
      settings: SourceProductName=IO Blocks
  wires:
  y/1 -> Data Type Conversion4/1
  Data Type Conversion4/1 -> Dio/1

== system RBCM_Model/HSD诊断分析子系统/HSDl片选执行单元1 ==
  y : Inport
  Bitwise AND2 : simulink/Logic and Bit Operations/Bitwise Operator  logicop=AND  UseBitMask=on  BitMask=bin2dec('00000001')  BitMaskRealWorld=Stored Integer
      settings: LibrarySourceBlock=|
      | simulink/Quick Insert/Logic and Bit
      | Operations/Bitwise AND
  Bitwise AND3 : simulink/Logic and Bit Operations/Bitwise Operator  logicop=AND  UseBitMask=on  BitMask=bin2dec('00000010')  BitMaskRealWorld=Stored Integer
      settings: LibrarySourceBlock=|
      | simulink/Quick Insert/Logic and Bit
      | Operations/Bitwise AND
  Data Type Conversion : DataTypeConversion  OutDataTypeStr=uint8  SaturateOnIntegerOverflow=off  RndMeth=Floor
  Data Type Conversion1 : DataTypeConversion  OutDataTypeStr=uint8  SaturateOnIntegerOverflow=off  RndMeth=Floor
  Dio : mbd_s32k3_io_library/Dio  api_func=Dio_WriteChannel  channel=RGBLED0_BLUE  channel_group=No channel groups configured  port=PTB_H  gpioSim=on  text=<binary blob, 15399 chars, not shown>
      settings: SourceProductName=IO Blocks
  Dio1 : mbd_s32k3_io_library/Dio  api_func=Dio_WriteChannel  channel=RGBLED0_BLUE  channel_group=No channel groups configured  port=PTB_H  gpioSim=on  text=<binary blob, 15399 chars, not shown>
      settings: SourceProductName=IO Blocks
  Shift Arithmetic1 : ArithShift  BitShiftNumber=1  BitShiftDirection=Right
  Shift Arithmetic2 : ArithShift  BitShiftDirection=Right
  wires:
  Shift Arithmetic1/1 -> Data Type Conversion1/1
  Bitwise AND2/1 -> Shift Arithmetic2/1
  Bitwise AND3/1 -> Shift Arithmetic1/1
  Shift Arithmetic2/1 -> Data Type Conversion/1
  y/1 -> Bitwise AND2/1, Bitwise AND3/1
  Data Type Conversion/1 -> Dio/1
  Data Type Conversion1/1 -> Dio1/1

== system RBCM_Model/HSD诊断分析子系统/HSDl片选执行单元2 ==
  y : Inport
  Bitwise AND2 : simulink/Logic and Bit Operations/Bitwise Operator  logicop=AND  UseBitMask=on  BitMask=bin2dec('00000001')  BitMaskRealWorld=Stored Integer
      settings: LibrarySourceBlock=|
      | simulink/Quick Insert/Logic and Bit
      | Operations/Bitwise AND
  Bitwise AND3 : simulink/Logic and Bit Operations/Bitwise Operator  logicop=AND  UseBitMask=on  BitMask=bin2dec('00000010')  BitMaskRealWorld=Stored Integer
      settings: LibrarySourceBlock=|
      | simulink/Quick Insert/Logic and Bit
      | Operations/Bitwise AND
  Data Type Conversion : DataTypeConversion  OutDataTypeStr=uint8  SaturateOnIntegerOverflow=off  RndMeth=Floor
  Data Type Conversion1 : DataTypeConversion  OutDataTypeStr=uint8  SaturateOnIntegerOverflow=off  RndMeth=Floor
  Dio : mbd_s32k3_io_library/Dio  api_func=Dio_WriteChannel  channel=RGBLED0_BLUE  channel_group=No channel groups configured  port=PTB_H  gpioSim=on  text=<binary blob, 15399 chars, not shown>
      settings: SourceProductName=IO Blocks
  Dio1 : mbd_s32k3_io_library/Dio  api_func=Dio_WriteChannel  channel=RGBLED0_BLUE  channel_group=No channel groups configured  port=PTB_H  gpioSim=on  text=<binary blob, 15399 chars, not shown>
      settings: SourceProductName=IO Blocks
  Shift Arithmetic1 : ArithShift  BitShiftNumber=1  BitShiftDirection=Right
  Shift Arithmetic2 : ArithShift  BitShiftDirection=Right
  wires:
  Data Type Conversion1/1 -> Dio1/1
  Data Type Conversion/1 -> Dio/1
  y/1 -> Bitwise AND3/1, Bitwise AND2/1
  Shift Arithmetic2/1 -> Data Type Conversion/1
  Bitwise AND3/1 -> Shift Arithmetic1/1
  Bitwise AND2/1 -> Shift Arithmetic2/1
  Shift Arithmetic1/1 -> Data Type Conversion1/1

== system RBCM_Model/HSD诊断分析子系统/HSDl片选执行单元3 ==
  y : Inport
  Bitwise AND2 : simulink/Logic and Bit Operations/Bitwise Operator  logicop=AND  UseBitMask=on  BitMask=bin2dec('00000001')  BitMaskRealWorld=Stored Integer
      settings: LibrarySourceBlock=|
      | simulink/Quick Insert/Logic and Bit
      | Operations/Bitwise AND
  Bitwise AND3 : simulink/Logic and Bit Operations/Bitwise Operator  logicop=AND  UseBitMask=on  BitMask=bin2dec('00000010')  BitMaskRealWorld=Stored Integer
      settings: LibrarySourceBlock=|
      | simulink/Quick Insert/Logic and Bit
      | Operations/Bitwise AND
  Data Type Conversion : DataTypeConversion  OutDataTypeStr=uint8  SaturateOnIntegerOverflow=off  RndMeth=Floor
  Data Type Conversion1 : DataTypeConversion  OutDataTypeStr=uint8  SaturateOnIntegerOverflow=off  RndMeth=Floor
  Dio : mbd_s32k3_io_library/Dio  api_func=Dio_WriteChannel  channel=RGBLED0_BLUE  channel_group=No channel groups configured  port=PTB_H  gpioSim=on  text=<binary blob, 15399 chars, not shown>
      settings: SourceProductName=IO Blocks
  Dio1 : mbd_s32k3_io_library/Dio  api_func=Dio_WriteChannel  channel=RGBLED0_BLUE  channel_group=No channel groups configured  port=PTB_H  gpioSim=on  text=<binary blob, 15399 chars, not shown>
      settings: SourceProductName=IO Blocks
  Shift Arithmetic1 : ArithShift  BitShiftNumber=1  BitShiftDirection=Right
  Shift Arithmetic2 : ArithShift  BitShiftDirection=Right
  wires:
  Data Type Conversion1/1 -> Dio1/1
  Data Type Conversion/1 -> Dio/1
  y/1 -> Bitwise AND3/1, Bitwise AND2/1
  Shift Arithmetic2/1 -> Data Type Conversion/1
  Bitwise AND3/1 -> Shift Arithmetic1/1
  Bitwise AND2/1 -> Shift Arithmetic2/1
  Shift Arithmetic1/1 -> Data Type Conversion1/1

== system RBCM_Model/HSD诊断分析子系统/HSDl片选执行单元4 ==
  y : Inport
  Bitwise AND2 : simulink/Logic and Bit Operations/Bitwise Operator  logicop=AND  UseBitMask=on  BitMask=bin2dec('00000001')  BitMaskRealWorld=Stored Integer
      settings: LibrarySourceBlock=|
      | simulink/Quick Insert/Logic and Bit
      | Operations/Bitwise AND
  Bitwise AND3 : simulink/Logic and Bit Operations/Bitwise Operator  logicop=AND  UseBitMask=on  BitMask=bin2dec('00000010')  BitMaskRealWorld=Stored Integer
      settings: LibrarySourceBlock=|
      | simulink/Quick Insert/Logic and Bit
      | Operations/Bitwise AND
  Data Type Conversion : DataTypeConversion  OutDataTypeStr=uint8  SaturateOnIntegerOverflow=off  RndMeth=Floor
  Data Type Conversion1 : DataTypeConversion  OutDataTypeStr=uint8  SaturateOnIntegerOverflow=off  RndMeth=Floor
  Dio : mbd_s32k3_io_library/Dio  api_func=Dio_WriteChannel  channel=RGBLED0_BLUE  channel_group=No channel groups configured  port=PTB_H  gpioSim=on  text=<binary blob, 15399 chars, not shown>
      settings: SourceProductName=IO Blocks
  Dio1 : mbd_s32k3_io_library/Dio  api_func=Dio_WriteChannel  channel=RGBLED0_BLUE  channel_group=No channel groups configured  port=PTB_H  gpioSim=on  text=<binary blob, 15399 chars, not shown>
      settings: SourceProductName=IO Blocks
  Shift Arithmetic1 : ArithShift  BitShiftNumber=1  BitShiftDirection=Right
  Shift Arithmetic2 : ArithShift  BitShiftDirection=Right
  wires:
  Shift Arithmetic1/1 -> Data Type Conversion1/1
  Bitwise AND2/1 -> Shift Arithmetic2/1
  Bitwise AND3/1 -> Shift Arithmetic1/1
  Shift Arithmetic2/1 -> Data Type Conversion/1
  y/1 -> Bitwise AND2/1, Bitwise AND3/1
  Data Type Conversion/1 -> Dio/1
  Data Type Conversion1/1 -> Dio1/1

== system RBCM_Model/HSD诊断分析子系统/HSDl片选执行单元5 ==
  y : Inport
  Bitwise AND2 : simulink/Logic and Bit Operations/Bitwise Operator  logicop=AND  UseBitMask=on  BitMask=bin2dec('00000001')  BitMaskRealWorld=Stored Integer
      settings: LibrarySourceBlock=|
      | simulink/Quick Insert/Logic and Bit
      | Operations/Bitwise AND
  Bitwise AND3 : simulink/Logic and Bit Operations/Bitwise Operator  logicop=AND  UseBitMask=on  BitMask=bin2dec('00000010')  BitMaskRealWorld=Stored Integer
      settings: LibrarySourceBlock=|
      | simulink/Quick Insert/Logic and Bit
      | Operations/Bitwise AND
  Data Type Conversion : DataTypeConversion  OutDataTypeStr=uint8  SaturateOnIntegerOverflow=off  RndMeth=Floor
  Data Type Conversion1 : DataTypeConversion  OutDataTypeStr=uint8  SaturateOnIntegerOverflow=off  RndMeth=Floor
  Dio : mbd_s32k3_io_library/Dio  api_func=Dio_WriteChannel  channel=RGBLED0_BLUE  channel_group=No channel groups configured  port=PTB_H  gpioSim=on  text=<binary blob, 15399 chars, not shown>
      settings: SourceProductName=IO Blocks
  Dio1 : mbd_s32k3_io_library/Dio  api_func=Dio_WriteChannel  channel=RGBLED0_BLUE  channel_group=No channel groups configured  port=PTB_H  gpioSim=on  text=<binary blob, 15399 chars, not shown>
      settings: SourceProductName=IO Blocks
  Shift Arithmetic1 : ArithShift  BitShiftNumber=1  BitShiftDirection=Right
  Shift Arithmetic2 : ArithShift  BitShiftDirection=Right
  wires:
  Data Type Conversion1/1 -> Dio1/1
  Data Type Conversion/1 -> Dio/1
  y/1 -> Bitwise AND3/1, Bitwise AND2/1
  Shift Arithmetic2/1 -> Data Type Conversion/1
  Bitwise AND3/1 -> Shift Arithmetic1/1
  Bitwise AND2/1 -> Shift Arithmetic2/1
  Shift Arithmetic1/1 -> Data Type Conversion1/1

== system RBCM_Model/HSD诊断分析子系统/Subsystem ==
  u1 : Inport
  Constant : Constant  Value=0xff  OutDataTypeStr=uint8
  Constant2 : Constant  Value=0  OutDataTypeStr=uint8
  Constant3 : Constant  OutDataTypeStr=uint8
  Constant4 : Constant  Value=2  OutDataTypeStr=uint8
  Gain : Gain  Gain=100
  Multiport Switch : MultiPortSwitch  DataPortOrder=Specify indices  DataPortIndices={0,5,90}  DataPortForDefault=Additional data port  DiagnosticForDefault=Warning  SaturateOnIntegerOverflow=off  InputSameDT=off
  u : Outport
  wires:
  u1/1 -> Gain/1
  Gain/1 -> Multiport Switch/1
  Multiport Switch/1 -> u/1
  Constant/1 -> Multiport Switch/5
  Constant2/1 -> Multiport Switch/2
  Constant3/1 -> Multiport Switch/3
  Constant4/1 -> Multiport Switch/4

== system RBCM_Model/HSD诊断分析子系统/Subsystem1 ==
  u1 : Inport
  Constant : Constant  Value=0xff  OutDataTypeStr=uint8
  Constant2 : Constant  Value=0  OutDataTypeStr=uint8
  Constant3 : Constant  OutDataTypeStr=uint8
  Constant4 : Constant  Value=2  OutDataTypeStr=uint8
  Gain : Gain  Gain=100
  Multiport Switch : MultiPortSwitch  DataPortOrder=Specify indices  DataPortIndices={0,5,290}  DataPortForDefault=Additional data port  DiagnosticForDefault=Warning  SaturateOnIntegerOverflow=off  InputSameDT=off
  u : Outport
  wires:
  Constant4/1 -> Multiport Switch/4
  Constant3/1 -> Multiport Switch/3
  Constant2/1 -> Multiport Switch/2
  Constant/1 -> Multiport Switch/5
  Multiport Switch/1 -> u/1
  Gain/1 -> Multiport Switch/1
  u1/1 -> Gain/1

== system RBCM_Model/HSD诊断分析子系统/Subsystem10 ==
  u1 : Inport
  Constant : Constant  Value=0xff  OutDataTypeStr=uint8
  Constant2 : Constant  Value=0  OutDataTypeStr=uint8
  Constant3 : Constant  OutDataTypeStr=uint8
  Constant4 : Constant  Value=2  OutDataTypeStr=uint8
  Gain : Gain  Gain=100
  Multiport Switch : MultiPortSwitch  DataPortOrder=Specify indices  DataPortIndices={0,5,290}  DataPortForDefault=Additional data port  DiagnosticForDefault=Warning  SaturateOnIntegerOverflow=off  InputSameDT=off
  u : Outport
  wires:
  Constant4/1 -> Multiport Switch/4
  Constant3/1 -> Multiport Switch/3
  Constant2/1 -> Multiport Switch/2
  Constant/1 -> Multiport Switch/5
  Multiport Switch/1 -> u/1
  Gain/1 -> Multiport Switch/1
  u1/1 -> Gain/1
